simulink model "dual_arm_control"  (Simulink 7.8)
settings: Solver=ode1  StartTime=0.0  StopTime=inf  FixedStep=0.001  RelTol=1e-3
undefined symbols (not defined in the file): HIL
libraries: quarc_library x48, simulink x26, dspmtrx3 x5
(part 1 of 2)
settings Model: Creator=danso  LastModifiedBy=danso  SimulationMode=external  ExtModeTrigDuration=5000
settings SolverCC: PositivePriorityOrder=on
settings RTWCC: SystemTargetFile=quarc_win64.tlc  TemplateMakefile=quarc_default_tmf  Description=QUARC Win64 Target  ProcessScript=quarc_win64_make_rtw_hook
settings STFCustomTargetCC: TargetPreCompLibLocation=C:\PROGRA~3\QUARC\lib\2011b\win64\release  SystemTargetFile=quarc_win64.tlc
settings GRTTargetCC: TargetPreCompLibLocation=C:\PROGRA~3\QUARC\lib\2011b\win64\release  ParMdlRefBuildCompliant=off  CompOptLevelCompliant=off  ConcurrentExecutionCompliant=off  MatFileLogging=off  ExtMode=on  ExtModeMexFile=quarc_comm

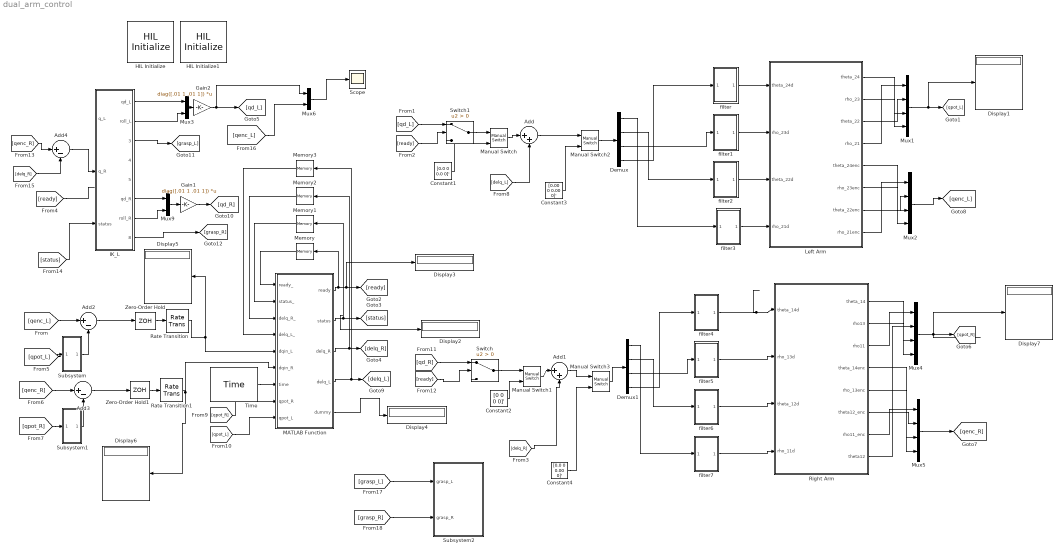
== system dual_arm_control ==
  Add : Sum  Inputs=|++
  Add1 : Sum  Inputs=|++
  Add2 : Sum  Inputs=|+-
  Add3 : Sum  Inputs=|+-
  Add4 : Sum  Inputs=|+-
  Constant1 : Constant  Value=[0.0 0 0.0 0]'
  Constant2 : Constant  Value=[0 0 0 0]'
  Constant3 : Constant  Value=[0.00 0 0.00 0]'
  Constant4 : Constant  Value=[0.0 0 0.00 0]'
  Demux : Demux
  Demux1 : Demux
  Display{1..7} (7 alike) : Display
  Gain1 : Gain  Gain=diag([.01 1 .01 1])  Multiplication=Matrix(K*u)
  Gain2 : Gain  Gain=diag([.01 1 .01 1])  Multiplication=Matrix(K*u)
  HIL Initialize : quarc_library/Data Acquisition/Generic/Configuration/HIL Initialize  Priority=-99  object_name=HIL-1  board_type=qpid_e  board_number=0  board_options=enc0_dir=0;enc0_filter=1;enc0_a=1;enc0_b=1;enc0_z=0;enc0_reload=0;enc1_dir=0;enc1_filter=1;enc1_a=1;enc1_b=1;enc1_z=0;enc1_reload=0;enc2_dir=0;enc2_filter=1;enc2_a=1;enc2_b=1;enc2_z=0;enc2_reload=0;enc3_dir=0;enc3_filter=1;enc3_a=1;enc3_b=1;enc3_z=0;enc3_reload=0;enc4_dir=0;enc4_filter=1;enc4_a=1;enc4_b=1;enc4_z=0;enc4_reload=0;enc5_dir=0;enc5_filter=1;enc5_a=1;enc5_b=1;enc5_z=0;enc5_reload=0;enc6_dir=0;enc6_filter=1;enc6_a=1;enc6_b=1;enc6_z=0;enc6_reload=0;enc7_dir=0;enc7_filter=1;enc7_a=1;enc7_b=1;enc7_z=0;enc7_reload=0;ext_int_polarity=0;fuse_polarity=0;convert_polarity=0;watchdog_polarity=0;ext_int_watchdog=0;fuse_watchdog=0;trig1_watchdog=0;watchdog_to_trig1=0;watchdog_to_trig2=0;counter_to_trig0=0;trigger_adcs=0;latch_on_adc=0;pwm_immediate=0  exclusive=off  active=off  hardware_clocks=[0:16]  clock_modes=[]  initial_clock_frequencies=[]  set_clock_params_at_start=off  set_clock_params_at_switch_in=off  set_clock_frequencies_at_start=off  set_clock_frequencies_at_switch_in=off  analog_input_channels=[0:7]  analog_input_maximums=10  analog_input_minimums=-10  set_analog_input_params_at_start=off  set_analog_input_params_at_switch_in=off  analog_output_channels=[0:7]  analog_output_maximums=10  analog_output_minimums=-10  initial_analog_outputs=[0]  final_analog_outputs=[0]  watchdog_analog_outputs=0  set_analog_output_params_at_start=off  set_analog_output_params_at_switch_in=off  set_analog_outputs_at_start=on  set_analog_outputs_at_switch_in=off  set_analog_outputs_at_terminate=on  set_analog_outputs_at_switch_out=off  set_analog_outputs_on_watchdog=off  digital_input_channels=[]  digital_output_channels=[0:31 46:47 40:45 55]  digital_output_configuration=[]  initial_digital_outputs=[1]  final_digital_outputs=[1]  watchdog_digital_outputs=[2]  set_digital_output_params_at_start=off  set_digital_output_params_at_switch_in=off  set_digital_outputs_at_start=on  set_digital_outputs_at_switch_in=off  set_digital_outputs_at_terminate=on  set_digital_outputs_at_switch_out=off  set_digital_outputs_on_watchdog=off  encoder_channels=[0:7]  quadrature=4  encoder_filter_frequency=40e6/1  initial_encoder_counts=[0]  set_encoder_params_at_start=on  set_encoder_params_at_switch_in=off  set_encoder_counts_at_start=on  set_encoder_counts_at_switch_in=off  pwm_channels=[0:7]  pwm_modes=0  pwm_frequency=40e6/4096  pwm_configuration=[0]  pwm_alignment=[0]  pwm_polarity=[1]  pwm_leading_deadband=[0]  pwm_trailing_deadband=[0]  initial_pwm_outputs=[0]  final_pwm_outputs=[0]  watchdog_pwm_outputs=[0]  set_pwm_params_at_start=on  set_pwm_params_at_switch_in=off  set_pwm_outputs_at_start=on  set_pwm_outputs_at_switch_in=off  set_pwm_outputs_at_terminate=on  set_pwm_outputs_at_switch_out=off  set_pwm_outputs_on_watchdog=off  other_output_channels=[]  initial_other_outputs=[]  final_other_outputs=[]  watchdog_other_outputs=[]  set_other_outputs_at_start=off  set_other_outputs_at_switch_in=off  set_other_outputs_at_terminate=off  set_other_outputs_at_switch_out=off  set_other_outputs_on_watchdog=off
  HIL Initialize1 : quarc_library/Data Acquisition/Generic/Configuration/HIL Initialize  Priority=-99  object_name=HIL-2  board_type=qpid  board_number=0  board_options=enc0_dir=0;enc0_filter=1;enc0_a=1;enc0_b=1;enc0_z=0;enc0_reload=0;enc1_dir=0;enc1_filter=1;enc1_a=1;enc1_b=1;enc1_z=0;enc1_reload=0;enc2_dir=0;enc2_filter=1;enc2_a=1;enc2_b=1;enc2_z=0;enc2_reload=0;enc3_dir=0;enc3_filter=1;enc3_a=1;enc3_b=1;enc3_z=0;enc3_reload=0;enc4_dir=0;enc4_filter=1;enc4_a=1;enc4_b=1;enc4_z=0;enc4_reload=0;enc5_dir=0;enc5_filter=1;enc5_a=1;enc5_b=1;enc5_z=0;enc5_reload=0;enc6_dir=0;enc6_filter=1;enc6_a=1;enc6_b=1;enc6_z=0;enc6_reload=0;enc7_dir=0;enc7_filter=1;enc7_a=1;enc7_b=1;enc7_z=0;enc7_reload=0;ext_int_polarity=0;fuse_polarity=0;convert_polarity=0;watchdog_polarity=0;ext_int_watchdog=0;fuse_watchdog=0;trig1_watchdog=0;watchdog_to_trig1=0;watchdog_to_trig2=0;counter_to_trig0=0;trigger_adcs=0;latch_on_adc=0;pwm_immediate=0  exclusive=off  active=off  hardware_clocks=[0:16]  clock_modes=[]  initial_clock_frequencies=[]  set_clock_params_at_start=off  set_clock_params_at_switch_in=off  set_clock_frequencies_at_start=off  set_clock_frequencies_at_switch_in=off  analog_input_channels=[0:7]  analog_input_maximums=10  analog_input_minimums=-10  set_analog_input_params_at_start=off  set_analog_input_params_at_switch_in=off  analog_output_channels=[0:7]  analog_output_maximums=10  analog_output_minimums=-10  initial_analog_outputs=[0]  final_analog_outputs=[0]  watchdog_analog_outputs=0  set_analog_output_params_at_start=off  set_analog_output_params_at_switch_in=off  set_analog_outputs_at_start=on  set_analog_outputs_at_switch_in=off  set_analog_outputs_at_terminate=on  set_analog_outputs_at_switch_out=off  set_analog_outputs_on_watchdog=off  digital_input_channels=[48:55]  digital_output_channels=[]  digital_output_configuration=[]  initial_digital_outputs=[1]  final_digital_outputs=[1]  watchdog_digital_outputs=[2]  set_digital_output_params_at_start=off  set_digital_output_params_at_switch_in=off  set_digital_outputs_at_start=on  set_digital_outputs_at_switch_in=off  set_digital_outputs_at_terminate=on  set_digital_outputs_at_switch_out=off  set_digital_outputs_on_watchdog=off  encoder_channels=[0:7]  quadrature=[4]  encoder_filter_frequency=40e6/1  initial_encoder_counts=[0]  set_encoder_params_at_start=on  set_encoder_params_at_switch_in=off  set_encoder_counts_at_start=on  set_encoder_counts_at_switch_in=off  pwm_channels=[0:7]  pwm_modes=0  pwm_frequency=40e6/4096  pwm_configuration=[0]  pwm_alignment=[0]  pwm_polarity=[1]  pwm_leading_deadband=[0]  pwm_trailing_deadband=[0]  initial_pwm_outputs=[0]  final_pwm_outputs=[0]  watchdog_pwm_outputs=[0]  set_pwm_params_at_start=on  set_pwm_params_at_switch_in=off  set_pwm_outputs_at_start=on  set_pwm_outputs_at_switch_in=off  set_pwm_outputs_at_terminate=on  set_pwm_outputs_at_switch_out=off  set_pwm_outputs_on_watchdog=off  other_output_channels=[]  initial_other_outputs=[]  final_other_outputs=[]  watchdog_other_outputs=[]  set_other_outputs_at_start=off  set_other_outputs_at_switch_in=off  set_other_outputs_at_terminate=off  set_other_outputs_at_switch_out=off  set_other_outputs_on_watchdog=off
  IK_L : Subsystem
  Left Arm : Subsystem
  MATLAB Function : MATLAB Function  TreatAsAtomicUnit=on
  Manual Switch{,1..3} (4 alike) : simulink/Signal Routing/Manual Switch  sw=1  action=0  varsize=off
  Memory : Memory
  Memory1 : Memory
  Memory2 : Memory  X0=[0 0 0 0 ]'
  Memory3 : Memory  X0=[0 0 0 0]'
  Mux{1..2,4..5} (4 alike) : Mux
  Mux3 : Mux  Inputs=[3 1]
  Mux6 : Mux  Inputs=2
  Mux9 : Mux  Inputs=[3 1]
  Rate Transition : RateTransition
  Rate Transition1 : RateTransition
  Right Arm : Subsystem
  Scope : Scope
      settings: YMin=-1.5  YMax=7.5
  Subsystem : Subsystem
  Subsystem1 : Subsystem
  Subsystem2 : Subsystem
  Switch : Switch  Criteria=u2 > Threshold
  Switch1 : Switch  Criteria=u2 > Threshold
  Time : quarc_library/Sources/Time/Time  sample_time=qc_get_step_size
  Zero-Order Hold : ZeroOrderHold  SampleTime=2
  Zero-Order Hold1 : ZeroOrderHold  SampleTime=2
  filter : Subsystem
  filter1 : Subsystem
  filter2 : Subsystem
  filter3 : Subsystem
  filter4 : Subsystem
  filter5 : Subsystem
  filter6 : Subsystem
  filter7 : Subsystem
  wires:
  IK_L/1(qd_L) -> Mux3/1
  Mux3/1 -> Gain2/1
  IK_L/2(roll_L) -> Mux3/2
  Mux9/1 -> Gain1/1
  IK_L/6(qd_R) -> Mux9/1
  IK_L/7(roll_R) -> Mux9/2
  [ready] -> ?
  ? -> IK_L/1(q_L)
  Demux/3 -> filter1/1(In1)
  Demux/4 -> filter/1(In1)
  Demux/2 -> filter2/1(In1)
  filter3/1(Out1) -> Left Arm/4(rho_21d)
  filter2/1(Out1) -> Left Arm/3(theta_22d)
  filter1/1(Out1) -> Left Arm/2(rho_23d)
  filter/1(Out1) -> Left Arm/1(theta_24d)
  Demux/1 -> filter3/1(In1)
  filter4/1(Out1) -> Right Arm/1(theta_14d)
  filter5/1(Out1) -> Right Arm/2(rho_13d)
  filter6/1(Out1) -> Right Arm/3(theta_12d)
  filter7/1(Out1) -> Right Arm/4(rho_11d)
  Mux5/1 -> [qenc_R]
  Mux4/1 -> [qpot_R], Display7/1
  Right Arm/3(rho11) -> Mux4/1
  Right Arm/2(rho13) -> Mux4/3
  Right Arm/1(theta_14) -> Mux4/4
  Right Arm/7(rho11_enc) -> Mux5/1
  Right Arm/6(theta12_enc) -> Mux5/2
  Right Arm/5(rho_13enc) -> Mux5/3
  Right Arm/4(theta_14enc) -> Mux5/4
  Left Arm/4(rho_21) -> Mux1/1
  Left Arm/3(theta_22) -> Mux1/2
  Left Arm/2(rho_23) -> Mux1/3
  Left Arm/1(theta_24) -> Mux1/4
  Left Arm/8(rho_21enc) -> Mux2/1
  Left Arm/7(theta_22enc) -> Mux2/2
  Left Arm/6(rho_23enc) -> Mux2/3
  Left Arm/5(theta_24enc) -> Mux2/4
  Demux1/4 -> filter4/1(In1)
  Demux1/2 -> filter6/1(In1)
  Demux1/1 -> filter7/1(In1)
  Mux1/1 -> [qpot_L], Display1/1
  Mux2/1 -> [qenc_L]
  Right Arm/8(theta12) -> Mux4/2
  Demux1/3 -> filter5/1(In1)
  Gain2/1 -> Mux6/1, [qd_L]
  Gain1/1 -> [qd_R]
  Constant2/1 -> Manual Switch1/2
  Constant1/1 -> Manual Switch/2
  [delq_L] -> Add/2
  [delq_R] -> Add1/2
  MATLAB Function/1(ready) -> Memory/1, [ready], Display3/1
  MATLAB Function/2(status) -> [status], Memory1/1, Display2/1
  Memory/1 -> MATLAB Function/1(ready_)
  Memory1/1 -> MATLAB Function/2(status_)
  Zero-Order Hold/1 -> Rate Transition/1
  [qenc_L] -> Add2/1
  [qpot_L] -> Subsystem/1(In1)
  Add2/1 -> Zero-Order Hold/1
  Rate Transition/1 -> Display5/1, MATLAB Function/5(dqin_L)
  Zero-Order Hold1/1 -> Rate Transition1/1
  [qenc_R] -> Add3/1
  [qpot_R] -> Subsystem1/1(In1)
  Add3/1 -> Zero-Order Hold1/1
  Rate Transition1/1 -> Display6/1, MATLAB Function/6(dqin_R)
  MATLAB Function/3(delq_R) -> [delq_R], Memory2/1
  MATLAB Function/4(delq_L) -> [delq_L], Memory3/1
  Time/1 -> MATLAB Function/7(time)
  MATLAB Function/5(dummy) -> Display4/1
  [qpot_R] -> MATLAB Function/8(qpot_R)
  [qpot_L] -> MATLAB Function/9(qpot_L)
  Memory2/1 -> MATLAB Function/3(delq_R_)
  Memory3/1 -> MATLAB Function/4(delq_L_)
  [ready] -> Switch/2
  Subsystem1/1(Out1) -> Add3/2
  [qd_R] -> Switch/1
  [status] -> IK_L/3(status)
  [qenc_R] -> Add4/1
  [delq_R] -> Add4/2
  Add4/1 -> IK_L/2(q_R)
  Subsystem/1(Out1) -> Add2/2
  Switch1/1 -> Manual Switch/1
  [qd_L] -> Switch1/1
  [ready] -> Switch1/2
  [qenc_L] -> Mux6/2
  Mux6/1 -> Scope/1
  Manual Switch/1 -> Add/1
  Manual Switch1/1 -> Add1/1
  Switch/1 -> Manual Switch1/1
  [grasp_L] -> Subsystem2/1(grasp_L)
  [grasp_R] -> Subsystem2/2(grasp_R)
  IK_L/3(grasp_L) -> [grasp_L]
  IK_L/8(grasp_R) -> [grasp_R]
  Manual Switch2/1 -> Demux/1
  Constant3/1 -> Manual Switch2/2
  Add/1 -> Manual Switch2/1
  Manual Switch3/1 -> Demux1/1
  Add1/1 -> Manual Switch3/1
  Constant4/1 -> Manual Switch3/2

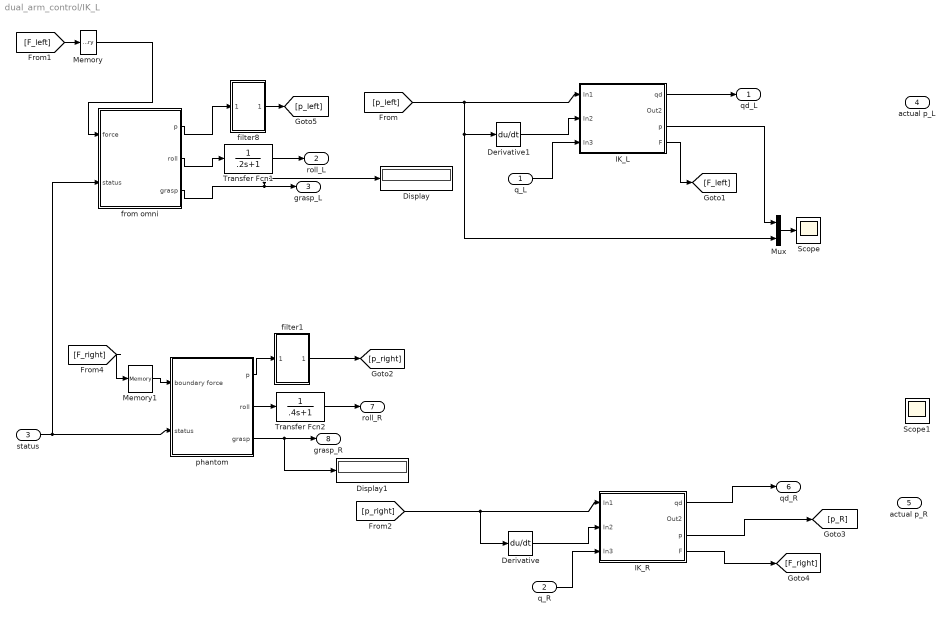
== system dual_arm_control/IK_L ==
  q_L : Inport
  q_R : Inport  Port=2
  status : Inport  Port=3
  Derivative : Derivative
  Derivative1 : Derivative
  Display : Display
  Display1 : Display
  IK_L : Subsystem
  IK_R : Subsystem
  Memory : Memory
  Memory1 : Memory
  Mux : Mux  Inputs=2
  Scope : Scope
      settings: YMin=-2  YMax=5.5
  Scope1 : Scope
      settings: YMin=-1.5  YMax=4  SaveName=ScopeData5
  Transfer Fcn1 : TransferFcn  Denominator=[.2 1]
  Transfer Fcn2 : TransferFcn  Denominator=[.4 1]
  filter1 : Subsystem
  filter8 : Subsystem
  from omni : Subsystem
  phantom : Subsystem
  qd_L : Outport
  roll_L : Outport  Port=2
  grasp_L : Outport  Port=3
  actual p_L : Outport  Port=4
  actual p_R : Outport  Port=5
  qd_R : Outport  Port=6
  roll_R : Outport  Port=7
  grasp_R : Outport  Port=8
  wires:
  from omni/1(p) -> filter8/1(In1)
  [F_left] -> Memory/1
  from omni/3(grasp) -> Display/1, grasp_L/1
  [p_left] -> Derivative1/1, Mux/2, IK_L/1(In1)
  Derivative1/1 -> IK_L/2(In2)
  IK_L/1(qd) -> qd_L/1
  IK_L/4(F) -> [F_left]
  Memory/1 -> from omni/1(force)
  phantom/1(p) -> filter1/1(In1)
  [F_right] -> Memory1/1
  phantom/2(roll) -> Transfer Fcn2/1
  phantom/3(grasp) -> grasp_R/1, Display1/1
  [p_right] -> Derivative/1, IK_R/1(In1)
  IK_R/4(F) -> [F_right]
  IK_R/1(qd) -> qd_R/1
  Derivative/1 -> IK_R/2(In2)
  from omni/2(roll) -> Transfer Fcn1/1
  Memory1/1 -> phantom/1(boundary force)
  filter1/1(Out1) -> [p_right]
  Transfer Fcn2/1 -> roll_R/1
  q_L/1 -> IK_L/3(In3)
  Mux/1 -> Scope/1
  IK_L/3(p) -> Mux/1
  status/1 -> phantom/2(status), from omni/2(status)
  IK_R/3(p) -> [p_R]
  q_R/1 -> IK_R/3(In3)
  Transfer Fcn1/1 -> roll_L/1
  filter8/1(Out1) -> [p_left]

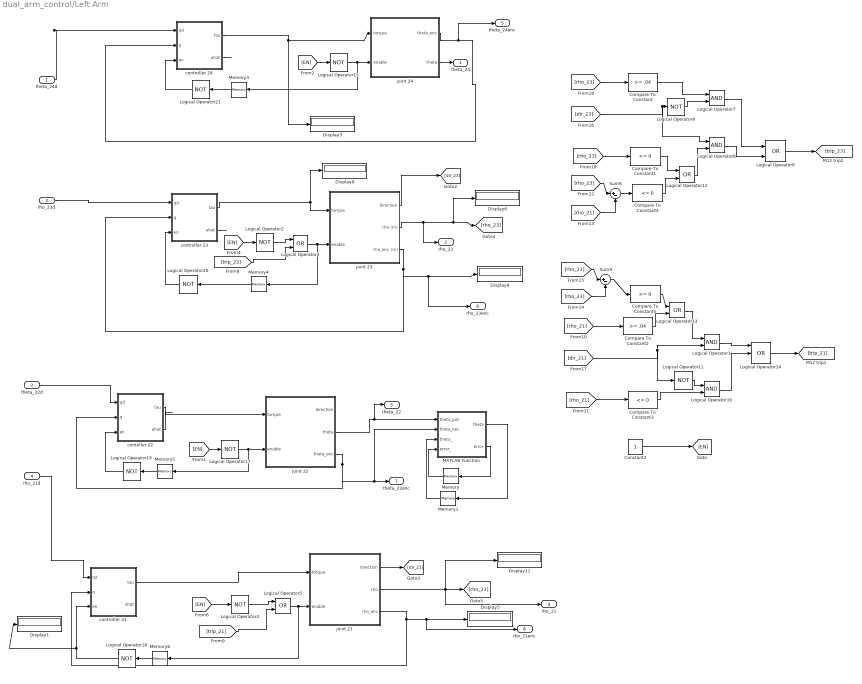
== system dual_arm_control/Left Arm ==
  theta_24d : Inport
  rho_23d : Inport  Port=2
  theta_22d : Inport  Port=3
  rho_21d : Inport  Port=4
  Compare To Constant : simulink/Logic and Bit Operations/Compare To Constant  relop=>=  const=.04  OutDataTypeStr=uint8
  Compare To Constant1 : simulink/Logic and Bit Operations/Compare To Constant  relop=<=  const=0  OutDataTypeStr=uint8
  Compare To Constant2 : simulink/Logic and Bit Operations/Compare To Constant  relop=>=  const=.04  OutDataTypeStr=uint8
  Compare To Constant3 : simulink/Logic and Bit Operations/Compare To Constant  relop=<=  const=0  OutDataTypeStr=uint8
  Compare To Constant4 : simulink/Logic and Bit Operations/Compare To Constant  relop=<=  const=0  OutDataTypeStr=uint8
  Compare To Constant5 : simulink/Logic and Bit Operations/Compare To Constant  relop=>=  const=0  OutDataTypeStr=uint8
  Constant2 : Constant
  Display{1,3,5..6,8..9,11} (7 alike) : Display
  Logical Operator{1,7..8,10} (4 alike) : Logic  AllPortsSameDT=off  OutDataTypeStr=boolean
  Logical Operator{2,4,9,11,15,17..21} (10 alike) : Logic  Operator=NOT  AllPortsSameDT=off  OutDataTypeStr=boolean
  Logical Operator{3,5..6,12..13} (5 alike) : Logic  Operator=OR  AllPortsSameDT=off  OutDataTypeStr=boolean
  Logical Operator14 : Logic  Operator=OR  Inputs=3  AllPortsSameDT=off  OutDataTypeStr=boolean
  MATLAB Function : MATLAB Function  TreatAsAtomicUnit=on
  Memory{,1,3..6} (6 alike) : Memory
  Sum8 : Sum  Inputs=|+-
  Sum9 : Sum  Inputs=|+-
  contoller 22 : Subsystem
  controller 21 : Subsystem
  controller 23 : Subsystem
  controller 24 : Subsystem
  joint 21 : Subsystem
  joint 22 : Subsystem
  joint 23 : Subsystem
  joint 24 : Subsystem
  theta_24 : Outport
  rho_23 : Outport  Port=2
  theta_22 : Outport  Port=3
  rho_21 : Outport  Port=4
  theta_24enc : Outport  Port=5
  rho_23enc : Outport  Port=6
  theta_22enc : Outport  Port=7
  rho_21enc : Outport  Port=8
  wires:
  Memory6/1 -> Logical Operator18/1
  Memory5/1 -> Logical Operator19/1
  [EN] -> Logical Operator4/1
  Logical Operator4/1 -> Logical Operator5/1
  [trip_21] -> Logical Operator5/2
  joint 21/2(rho) -> [rho_21], Display11/1, rho_21/1
  joint 22/3(theta_enc) -> contoller 22/2(q), theta_22enc/1, MATLAB Function/2(theta_enc)
  contoller 22/1(tau) -> joint 22/1(torque)
  Logical Operator17/1 -> joint 22/2(enable), Memory5/1
  [EN] -> Logical Operator17/1
  joint 21/1(direction) -> [dir_21]
  Logical Operator5/1 -> joint 21/2(enable), Memory6/1
  joint 21/3(rho_enc) -> Display5/1, rho_21enc/1, controller 21/2(q)
  joint 24/1(theta_enc) -> controller 24/2(q), theta_24enc/1
  controller 24/1(tau) -> Display3/1, joint 24/1(torque)
  [EN] -> Logical Operator2/1
  [trip_23] -> Logical Operator3/2
  Logical Operator2/1 -> Logical Operator3/1
  joint 23/1(direction) -> [dir_23]
  Logical Operator3/1 -> joint 23/2(enable), Memory4/1
  theta_24d/1 -> controller 24/1(qd)
  joint 23/2(rho (m)) -> [rho_23], Display6/1, rho_23/1
  joint 23/3(rho_enc (m)) -> controller 23/2(q), Display8/1, rho_23enc/1
  controller 23/1(tau) -> Display9/1, joint 23/1(torque)
  [EN] -> Logical Operator15/1
  Logical Operator15/1 -> joint 24/2(enable), Memory3/1
  Memory3/1 -> Logical Operator21/1
  Memory4/1 -> Logical Operator20/1
  controller 24/2(ahat) -> ?
  joint 24/2(theta) -> theta_24/1
  rho_23d/1 -> controller 23/1(qd)
  controller 23/2(ahat) -> ?
  theta_22d/1 -> contoller 22/1(qd)
  contoller 22/2(ahat) -> ?
  rho_21d/1 -> controller 21/1(qd)
  Logical Operator6/1 -> [trip_23]
  [dir_23] -> Logical Operator8/1, Logical Operator9/1
  Compare To Constant/1 -> Logical Operator7/1
  [rho_23] -> Compare To Constant1/1
  Logical Operator7/1 -> Logical Operator6/1
  Logical Operator8/1 -> Logical Operator6/2
  Logical Operator9/1 -> Logical Operator7/2
  [rho_23] -> Sum8/1
  [rho_21] -> Sum8/2
  Sum8/1 -> Compare To Constant4/1
  Compare To Constant4/1 -> Logical Operator12/2
  Compare To Constant1/1 -> Logical Operator12/1
  Logical Operator12/1 -> Logical Operator8/2
  [dir_21] -> Logical Operator11/1, Logical Operator1/2
  Compare To Constant3/1 -> Logical Operator10/2
  Logical Operator11/1 -> Logical Operator10/1
  [rho_21] -> Compare To Constant2/1
  [rho_21] -> Compare To Constant3/1
  Logical Operator13/1 -> Logical Operator1/1
  Compare To Constant2/1 -> Logical Operator13/2
  Sum9/1 -> Compare To Constant5/1
  [rho_21] -> Sum9/1
  [rho_23] -> Sum9/2
  Compare To Constant5/1 -> Logical Operator13/1
  Logical Operator1/1 -> Logical Operator14/1
  Logical Operator10/1 -> Logical Operator14/2
  Logical Operator14/1 -> [trip_21]
  Constant2/1 -> [EN]
  controller 21/1(tau) -> joint 21/1(torque)
  Logical Operator18/1 -> controller 21/3(en), Display1/1
  Logical Operator19/1 -> contoller 22/3(en)
  Logical Operator20/1 -> controller 23/3(en)
  Logical Operator21/1 -> controller 24/3(en)
  [rho_23] -> Compare To Constant/1
  Memory/1 -> MATLAB Function/4(error_)
  MATLAB Function/2(error) -> Memory/1
  MATLAB Function/1(theta) -> Memory1/1
  Memory1/1 -> MATLAB Function/3(theta_)
  joint 22/2(theta) -> MATLAB Function/1(theta_pot), theta_22/1

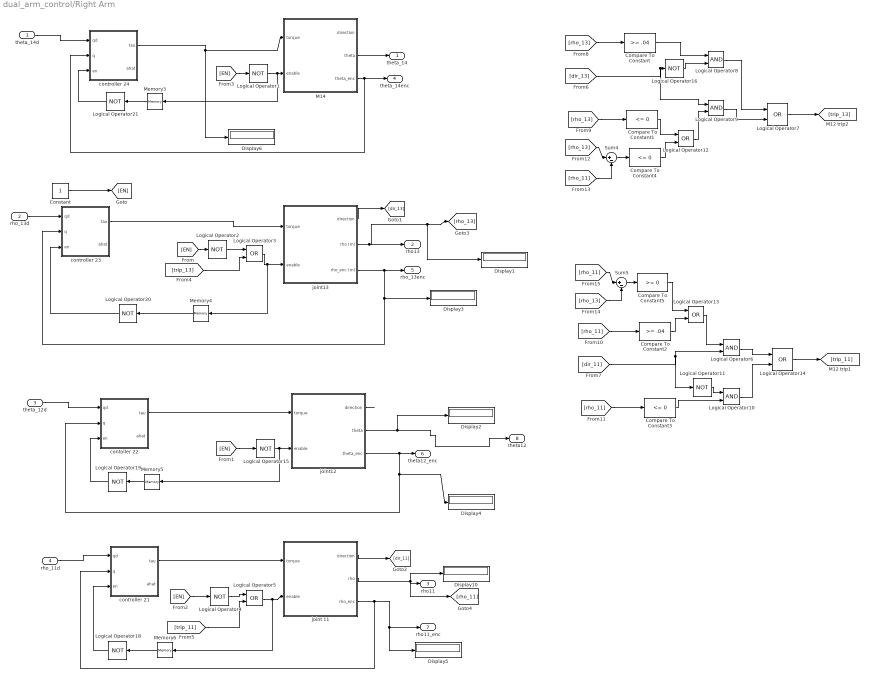
== system dual_arm_control/Right Arm ==
  theta_14d : Inport
  rho_13d : Inport  Port=2
  theta_12d : Inport  Port=3
  rho_11d : Inport  Port=4
  Compare To Constant : simulink/Logic and Bit Operations/Compare To Constant  relop=>=  const=.04  OutDataTypeStr=uint8
  Compare To Constant1 : simulink/Logic and Bit Operations/Compare To Constant  relop=<=  const=0  OutDataTypeStr=uint8
  Compare To Constant2 : simulink/Logic and Bit Operations/Compare To Constant  relop=>=  const=.04  OutDataTypeStr=uint8
  Compare To Constant3 : simulink/Logic and Bit Operations/Compare To Constant  relop=<=  const=0  OutDataTypeStr=uint8
  Compare To Constant4 : simulink/Logic and Bit Operations/Compare To Constant  relop=<=  const=0  OutDataTypeStr=uint8
  Compare To Constant5 : simulink/Logic and Bit Operations/Compare To Constant  relop=>=  const=0  OutDataTypeStr=uint8
  Constant : Constant
  Display{1..6,10} (7 alike) : Display
  Logical Operator{1..2,4,11,15..16,18..21} (10 alike) : Logic  Operator=NOT  AllPortsSameDT=off  OutDataTypeStr=boolean
  Logical Operator{6,8..10} (4 alike) : Logic  AllPortsSameDT=off  OutDataTypeStr=boolean
  Logical Operator{3,5,7,12..14} (6 alike) : Logic  Operator=OR  AllPortsSameDT=off  OutDataTypeStr=boolean
  M14 : Subsystem
  Memory{3..6} (4 alike) : Memory
  Sum4 : Sum  Inputs=|+-
  Sum5 : Sum  Inputs=|+-
  contoller 22 : Subsystem
  controller 21 : Subsystem
  controller 23 : Subsystem
  controller 24 : Subsystem
  joint 11 : Subsystem
  joint12 : Subsystem
  joint13 : Subsystem
  theta_14 : Outport
  rho13 : Outport  Port=2
  rho11 : Outport  Port=3
  theta_14enc : Outport  Port=4
  rho_13enc : Outport  Port=5
  theta12_enc : Outport  Port=6
  rho11_enc : Outport  Port=7
  theta12 : Outport  Port=8
  wires:
  Constant/1 -> [EN]
  [EN] -> Logical Operator2/1
  Logical Operator3/1 -> joint13/2(enable), Memory4/1
  [trip_13] -> Logical Operator3/2
  Logical Operator2/1 -> Logical Operator3/1
  joint13/1(direction) -> [dir_13]
  controller 23/1(tau) -> joint13/1(torque)
  joint13/2(rho (m)) -> rho13/1, [rho_13], Display1/1
  joint13/3(rho_enc (m)) -> Display3/1, controller 23/2(q), rho_13enc/1
  Memory4/1 -> Logical Operator20/1
  Logical Operator20/1 -> controller 23/3(en)
  [EN] -> Logical Operator15/1
  Logical Operator15/1 -> joint12/2(enable), Memory5/1
  joint12/3(theta_enc) -> contoller 22/2(q), Display4/1, theta12_enc/1
  joint12/2(theta) -> Display2/1, theta12/1
  Memory5/1 -> Logical Operator19/1
  Logical Operator19/1 -> contoller 22/3(en)
  contoller 22/1(tau) -> joint12/1(torque)
  [trip_11] -> Logical Operator5/2
  Logical Operator4/1 -> Logical Operator5/1
  [EN] -> Logical Operator4/1
  Logical Operator5/1 -> joint 11/2(enable), Memory6/1
  joint 11/1(direction) -> [dir_11]
  joint 11/3(rho_enc) -> Display5/1, rho11_enc/1, controller 21/2(q)
  joint 11/2(rho) -> rho11/1, Display10/1, [rho_11]
  controller 21/1(tau) -> joint 11/1(torque)
  Memory6/1 -> Logical Operator18/1
  Logical Operator18/1 -> controller 21/3(en)
  M14/2(theta) -> theta_14/1
  controller 24/1(tau) -> Display6/1, M14/1(torque)
  [EN] -> Logical Operator1/1
  Logical Operator1/1 -> Memory3/1, M14/2(enable)
  Memory3/1 -> Logical Operator21/1
  M14/3(theta_enc) -> controller 24/2(q), theta_14enc/1
  Logical Operator21/1 -> controller 24/3(en)
  theta_14d/1 -> controller 24/1(qd)
  rho_13d/1 -> controller 23/1(qd)
  theta_12d/1 -> contoller 22/1(qd)
  rho_11d/1 -> controller 21/1(qd)
  joint12/1(direction) -> ?
  Logical Operator7/1 -> [trip_13]
  [dir_13] -> Logical Operator9/1, Logical Operator16/1
  Compare To Constant/1 -> Logical Operator8/1
  [rho_13] -> Compare To Constant/1
  [rho_13] -> Compare To Constant1/1
  [dir_11] -> Logical Operator11/1, Logical Operator6/2
  Compare To Constant3/1 -> Logical Operator10/2
  Logical Operator11/1 -> Logical Operator10/1
  [rho_11] -> Compare To Constant2/1
  [rho_11] -> Compare To Constant3/1
  Logical Operator8/1 -> Logical Operator7/1
  Logical Operator9/1 -> Logical Operator7/2
  Logical Operator16/1 -> Logical Operator8/2
  [rho_13] -> Sum4/1
  [rho_11] -> Sum4/2
  Sum4/1 -> Compare To Constant4/1
  Compare To Constant4/1 -> Logical Operator12/2
  Compare To Constant1/1 -> Logical Operator12/1
  Logical Operator12/1 -> Logical Operator9/2
  Logical Operator13/1 -> Logical Operator6/1
  Compare To Constant2/1 -> Logical Operator13/2
  Sum5/1 -> Compare To Constant5/1
  [rho_11] -> Sum5/1
  [rho_13] -> Sum5/2
  Compare To Constant5/1 -> Logical Operator13/1
  Logical Operator6/1 -> Logical Operator14/1
  Logical Operator10/1 -> Logical Operator14/2
  Logical Operator14/1 -> [trip_11]

== system dual_arm_control/Subsystem ==
  In1 : Inport
  Demux2 : Demux
  Mux6 : Mux
  Transfer Fcn{,1..3} (4 alike) : TransferFcn  Denominator=[1 1]
  Out1 : Outport
  wires:
  Transfer Fcn3/1 -> Mux6/1
  Transfer Fcn2/1 -> Mux6/2
  Transfer Fcn1/1 -> Mux6/3
  Transfer Fcn/1 -> Mux6/4
  Demux2/1 -> Transfer Fcn3/1
  Demux2/2 -> Transfer Fcn2/1
  Demux2/3 -> Transfer Fcn1/1
  Demux2/4 -> Transfer Fcn/1
  Mux6/1 -> Out1/1
  In1/1 -> Demux2/1

== system dual_arm_control/Subsystem1 ==
  In1 : Inport
  Demux2 : Demux
  Mux6 : Mux
  Transfer Fcn{,1..3} (4 alike) : TransferFcn  Denominator=[1 1]
  Out1 : Outport
  wires:
  Transfer Fcn3/1 -> Mux6/1
  Transfer Fcn2/1 -> Mux6/2
  Transfer Fcn1/1 -> Mux6/3
  Transfer Fcn/1 -> Mux6/4
  Demux2/1 -> Transfer Fcn3/1
  Demux2/2 -> Transfer Fcn2/1
  Demux2/3 -> Transfer Fcn1/1
  Demux2/4 -> Transfer Fcn/1
  Mux6/1 -> Out1/1
  In1/1 -> Demux2/1

== system dual_arm_control/Subsystem2 ==
  grasp_L : Inport
  grasp_R : Inport  Port=2
  Constant : Constant  Value=9.2
  Constant1 : Constant  Value=6
  Constant2 : Constant  Value=9.5
  Constant3 : Constant  Value=6.5
  Demux : Demux  Outputs=3
  Demux1 : Demux  Outputs=3
  Display3 : Display
  Display5 : Display
  E1-1 : Subsystem
  E1-2 : Subsystem
  MATLAB Function : MATLAB Function  TreatAsAtomicUnit=on
  MATLAB Function1 : MATLAB Function  TreatAsAtomicUnit=on
  Mux : Mux  Inputs=3
  Mux1 : Mux  Inputs=3
  Subsystem : Subsystem
  wires:
  E1-1/1(Out1) -> Display3/1, MATLAB Function/2(pos)
  E1-2/1(Out1) -> Display5/1, MATLAB Function1/2(pos)
  MATLAB Function/1(dir) -> Mux/1
  MATLAB Function/2(en) -> Mux/2
  MATLAB Function/3(pwm) -> Mux/3
  MATLAB Function1/1(dir) -> Mux1/1
  MATLAB Function1/2(en) -> Mux1/2
  MATLAB Function1/3(pwm) -> Mux1/3
  Mux/1 -> Demux/1
  Demux/1 -> Subsystem/1(DIR_1)
  Demux/2 -> Subsystem/2(EN_1)
  Demux/3 -> Subsystem/3(PWM_1)
  Mux1/1 -> Demux1/1
  Demux1/1 -> Subsystem/4(DIR_2)
  Demux1/2 -> Subsystem/5(EN_2)
  Demux1/3 -> Subsystem/6(PWM_2)
  grasp_L/1 -> MATLAB Function/1(u)
  grasp_R/1 -> MATLAB Function1/1(u)
  Constant/1 -> MATLAB Function/3(pmax)
  Constant1/1 -> MATLAB Function/4(pmin)
  Constant2/1 -> MATLAB Function1/3(pmax)
  Constant3/1 -> MATLAB Function1/4(pmin)

== system dual_arm_control/filter ==
  In1 : Inport
  Memory : Memory
  filter : MATLAB Function  TreatAsAtomicUnit=on
  Out1 : Outport
  wires:
  filter/1(y) -> Memory/1, Out1/1
  Memory/1 -> filter/2(u_)
  In1/1 -> filter/1(u)

== system dual_arm_control/filter1 ==
  In1 : Inport
  Memory : Memory
  filter : MATLAB Function  TreatAsAtomicUnit=on
  Out1 : Outport
  wires:
  filter/1(y) -> Memory/1, Out1/1
  Memory/1 -> filter/2(u_)
  In1/1 -> filter/1(u)

== system dual_arm_control/filter2 ==
  In1 : Inport
  Memory : Memory
  filter : MATLAB Function  TreatAsAtomicUnit=on
  Out1 : Outport
  wires:
  filter/1(y) -> Memory/1, Out1/1
  Memory/1 -> filter/2(u_)
  In1/1 -> filter/1(u)

== system dual_arm_control/filter3 ==
  In1 : Inport
  Memory : Memory
  filter : MATLAB Function  TreatAsAtomicUnit=on
  Out1 : Outport
  wires:
  filter/1(y) -> Memory/1, Out1/1
  Memory/1 -> filter/2(u_)
  In1/1 -> filter/1(u)

== system dual_arm_control/filter4 ==
  In1 : Inport
  Memory : Memory
  filter : MATLAB Function  TreatAsAtomicUnit=on
  Out1 : Outport
  wires:
  filter/1(y) -> Memory/1, Out1/1
  Memory/1 -> filter/2(u_)
  In1/1 -> filter/1(u)

== system dual_arm_control/filter5 ==
  In1 : Inport
  Memory : Memory
  filter : MATLAB Function  TreatAsAtomicUnit=on
  Out1 : Outport
  wires:
  filter/1(y) -> Memory/1, Out1/1
  Memory/1 -> filter/2(u_)
  In1/1 -> filter/1(u)

== system dual_arm_control/filter6 ==
  In1 : Inport
  Memory : Memory
  filter : MATLAB Function  TreatAsAtomicUnit=on
  Out1 : Outport
  wires:
  filter/1(y) -> Memory/1, Out1/1
  Memory/1 -> filter/2(u_)
  In1/1 -> filter/1(u)

== system dual_arm_control/filter7 ==
  In1 : Inport
  Memory : Memory
  filter : MATLAB Function  TreatAsAtomicUnit=on
  Out1 : Outport
  wires:
  filter/1(y) -> Memory/1, Out1/1
  Memory/1 -> filter/2(u_)
  In1/1 -> filter/1(u)

== system dual_arm_control/IK_L/IK_L ==
  In1 : Inport
  In2 : Inport  Port=2
  In3 : Inport  Port=3
  Display : Display
  IK : MATLAB Function  TreatAsAtomicUnit=on
  Integrator : Integrator
  Memory1 : Memory  X0=[0 0 0]'
  Memory3 : Memory
  Memory4 : Memory
  qd : Outport
  Out2 : Outport  Port=2
  p : Outport  Port=3
  F : Outport  Port=4
  wires:
  IK/1(q) -> Memory1/1
  IK/5(F) -> F/1
  IK/6(k) -> Memory3/1
  Memory3/1 -> IK/4(k_)
  IK/3(qdot) -> Integrator/1
  IK/2(qm) -> qd/1, Display/1
  IK/7(r) -> Memory4/1
  Memory4/1 -> IK/5(r_)
  In1/1 -> IK/2(pd)
  Integrator/1 -> Out2/1
  In2/1 -> IK/3(pd_d)
  IK/4(p) -> p/1
  Memory1/1 -> IK/1(q_)

== system dual_arm_control/IK_L/IK_R ==
  In1 : Inport
  In2 : Inport  Port=2
  In3 : Inport  Port=3
  Display : Display
  IK : MATLAB Function  TreatAsAtomicUnit=on
  Integrator : Integrator
  Memory1 : Memory  X0=[0 0 0]'
  Memory3 : Memory
  Memory4 : Memory
  qd : Outport
  Out2 : Outport  Port=2
  p : Outport  Port=3
  F : Outport  Port=4
  wires:
  IK/1(q) -> Memory1/1
  IK/5(F) -> F/1
  IK/6(k) -> Memory3/1
  Memory3/1 -> IK/4(k_)
  IK/3(qdot) -> Integrator/1
  IK/2(qm) -> qd/1, Display/1
  IK/7(r) -> Memory4/1
  Memory4/1 -> IK/5(r_)
  In1/1 -> IK/2(pd)
  Integrator/1 -> Out2/1
  In2/1 -> IK/3(pd_d)
  IK/4(p) -> p/1
  Memory1/1 -> IK/1(q_)

== system dual_arm_control/IK_L/filter1 ==
  In1 : Inport
  Demux : Demux  Outputs=3
  Mux : Mux  Inputs=3
  Transfer Fcn : TransferFcn  Denominator=[.4 1]
  Transfer Fcn1 : TransferFcn  Denominator=[.4 1]
  Transfer Fcn2 : TransferFcn  Denominator=[.4 1]
  Out1 : Outport
  wires:
  Transfer Fcn/1 -> Mux/1
  Transfer Fcn1/1 -> Mux/2
  Transfer Fcn2/1 -> Mux/3
  Demux/1 -> Transfer Fcn/1
  Demux/2 -> Transfer Fcn1/1
  Demux/3 -> Transfer Fcn2/1
  Mux/1 -> Out1/1
  In1/1 -> Demux/1

== system dual_arm_control/IK_L/filter8 ==
  In1 : Inport
  Demux : Demux  Outputs=3
  Mux : Mux  Inputs=3
  Transfer Fcn : TransferFcn  Denominator=[.5 1]
  Transfer Fcn1 : TransferFcn  Denominator=[.5 1]
  Transfer Fcn2 : TransferFcn  Denominator=[.5 1]
  Out1 : Outport
  wires:
  Transfer Fcn/1 -> Mux/1
  Transfer Fcn1/1 -> Mux/2
  Transfer Fcn2/1 -> Mux/3
  Demux/1 -> Transfer Fcn/1
  Demux/2 -> Transfer Fcn1/1
  Demux/3 -> Transfer Fcn2/1
  Mux/1 -> Out1/1
  In1/1 -> Demux/1

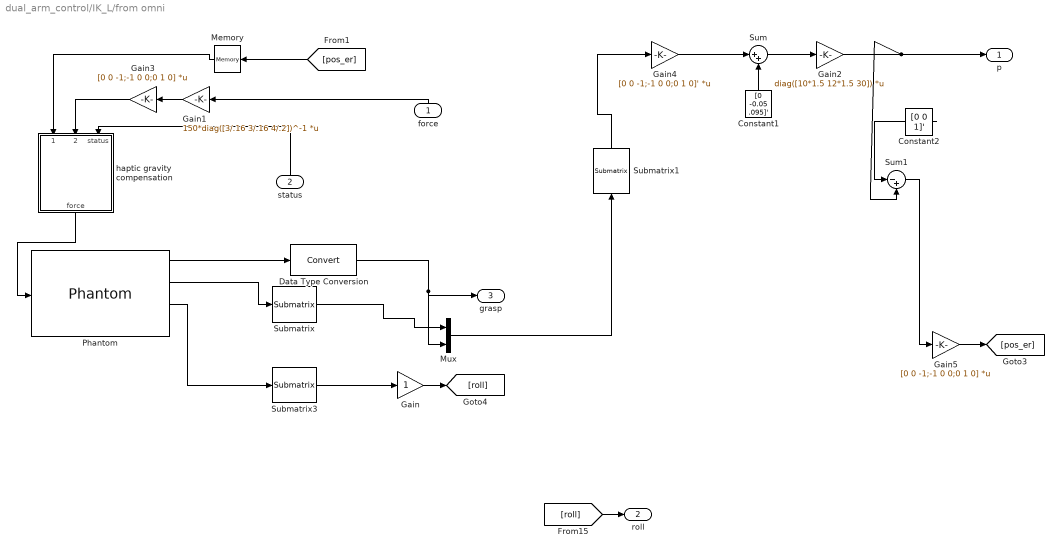
== system dual_arm_control/IK_L/from omni ==
  force : Inport
  status : Inport  Port=2
  Constant1 : Constant  Value=[0 -0.05 .095]'
  Constant2 : Constant  Value=[0 0 1]'
  Data Type Conversion : DataTypeConversion
  Gain : Gain
  Gain1 : Gain  Gain=150*diag([3/.16 3/.16 4/.2])^-1  Multiplication=Matrix(K*u)
  Gain2 : Gain  Gain=diag([10*1.5 12*1.5 30])  Multiplication=Matrix(K*u)
  Gain3 : Gain  Gain=[0 0 -1;-1 0 0;0 1 0]  Multiplication=Matrix(K*u)
  Gain4 : Gain  Gain=[0 0 -1;-1 0 0;0 1 0]'  Multiplication=Matrix(K*u)
  Gain5 : Gain  Gain=[0 0 -1;-1 0 0;0 1 0]  Multiplication=Matrix(K*u)
  Memory : Memory
  Mux : Mux  Inputs=2
  Phantom : quarc_library/Devices/Third-Party/SensAble/Phantom/Phantom  device_name=CIGITI omni  output_type=Positions and Gimbal Angles  input_type=Cartesian space  velocity_limit_option=on  velocity_limit=1200  is_7dof=off  sample_time=-1
      settings: AttributesFormatString=(%<device_name>)
  Submatrix : dspmtrx3/Submatrix  RowSpan=Range of rows  RowStartMode=First  RowStartIndex=1  RowEndMode=Index  RowEndIndex=3  ColSpan=Range of columns  ColStartMode=First  ColStartIndex=1  ColEndMode=Last  ColEndIndex=1
  Submatrix1 : dspmtrx3/Submatrix  RowSpan=Range of rows  RowStartMode=First  RowStartIndex=1  RowEndMode=Index  RowEndIndex=3  ColSpan=Range of columns  ColStartMode=First  ColStartIndex=1  ColEndMode=Last  ColEndIndex=1
  Submatrix3 : dspmtrx3/Submatrix  RowSpan=Range of rows  RowStartMode=Last  RowStartIndex=1  RowEndMode=Index  RowEndIndex=3  ColSpan=All columns  ColStartMode=First  ColStartIndex=1  ColEndMode=Last  ColEndIndex=1
  Sum : Sum  Inputs=|++
  Sum1 : Sum  Inputs=|-+
  haptic gravity compensation : Subsystem
  p : Outport
  roll : Outport  Port=2
  grasp : Outport  Port=3
  wires:
  Phantom/2 -> Submatrix/1
  Submatrix/1 -> Mux/1
  Phantom/1 -> Data Type Conversion/1
  Data Type Conversion/1 -> Mux/2, grasp/1
  Submatrix1/1 -> Gain4/1
  Constant1/1 -> Sum/2
  Sum/1 -> Gain2/1
  Gain4/1 -> Sum/1
  Mux/1 -> Submatrix1/1
  Submatrix3/1 -> Gain/1
  Phantom/3 -> Submatrix3/1
  Gain/1 -> [roll]
  Gain2/1 -> p/1, Sum1/2
  [roll] -> roll/1
  force/1 -> Gain1/1
  Memory/1 -> haptic gravity compensation/1(position)
  Gain1/1 -> Gain3/1
  Gain3/1 -> haptic gravity compensation/2(boundary force)
  [pos_er] -> Memory/1
  status/1 -> haptic gravity compensation/3(status)
  haptic gravity compensation/1(force) -> Phantom/1
  Sum1/1 -> Gain5/1
  Gain5/1 -> [pos_er]
  Constant2/1 -> Sum1/1

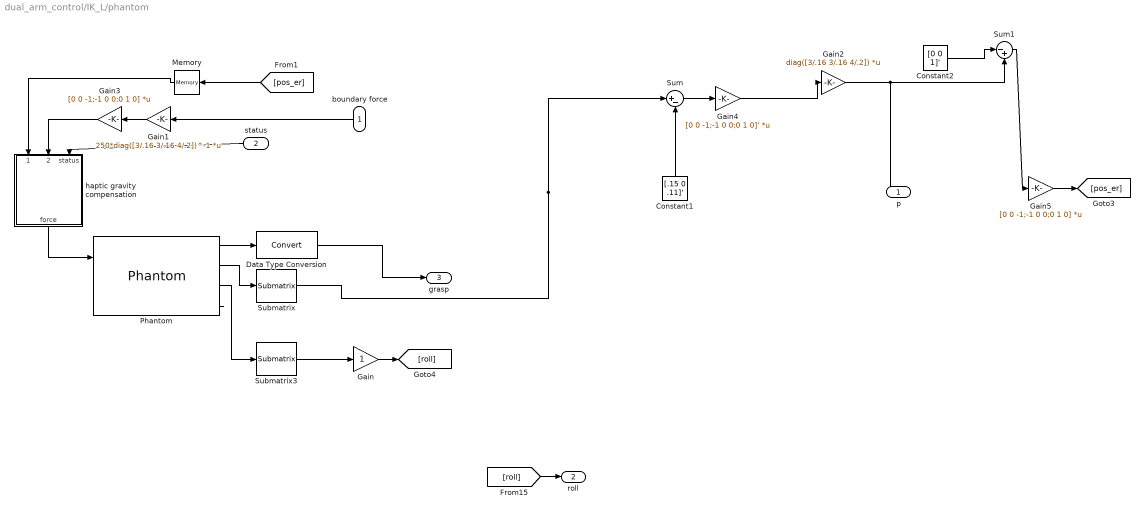
== system dual_arm_control/IK_L/phantom ==
  boundary force : Inport
  status : Inport  Port=2
  Constant1 : Constant  Value=[.15 0 .11]'
  Constant2 : Constant  Value=[0 0 1]'
  Data Type Conversion : DataTypeConversion
  Gain : Gain
  Gain1 : Gain  Gain=250*diag([3/.16 3/.16 4/.2])^-1  Multiplication=Matrix(K*u)
  Gain2 : Gain  Gain=diag([3/.16 3/.16 4/.2])  Multiplication=Matrix(K*u)
  Gain3 : Gain  Gain=[0 0 -1;-1 0 0;0 1 0]  Multiplication=Matrix(K*u)
  Gain4 : Gain  Gain=[0 0 -1;-1 0 0;0 1 0]'  Multiplication=Matrix(K*u)
  Gain5 : Gain  Gain=[0 0 -1;-1 0 0;0 1 0]  Multiplication=Matrix(K*u)
  Memory : Memory
  Phantom : quarc_library/Devices/Third-Party/SensAble/Phantom/Phantom  device_name=Default PHANToM  output_type=Positions and Gimbal Angles  input_type=Cartesian space  velocity_limit_option=on  velocity_limit=1200  is_7dof=off  sample_time=-1
      settings: AttributesFormatString=(%<device_name>)
  Submatrix : dspmtrx3/Submatrix  RowSpan=Range of rows  RowStartMode=First  RowStartIndex=1  RowEndMode=Index  RowEndIndex=3  ColSpan=Range of columns  ColStartMode=First  ColStartIndex=1  ColEndMode=Last  ColEndIndex=1
  Submatrix3 : dspmtrx3/Submatrix  RowSpan=Range of rows  RowStartMode=Last  RowStartIndex=1  RowEndMode=Index  RowEndIndex=3  ColSpan=All columns  ColStartMode=First  ColStartIndex=1  ColEndMode=Last  ColEndIndex=1
  Sum : Sum  Inputs=|+-
  Sum1 : Sum  Inputs=|-+
  haptic gravity compensation : Subsystem
  p : Outport
  roll : Outport  Port=2
  grasp : Outport  Port=3
  wires:
  Phantom/2 -> Submatrix/1
  Submatrix/1 -> Sum/1
  Phantom/1 -> Data Type Conversion/1
  Data Type Conversion/1 -> grasp/1
  Submatrix3/1 -> Gain/1
  Phantom/3 -> Submatrix3/1
  Gain/1 -> [roll]
  Gain2/1 -> p/1, Sum1/2
  Phantom/4 -> ?
  [roll] -> roll/1
  haptic gravity compensation/1(force) -> Phantom/1
  boundary force/1 -> Gain1/1
  Memory/1 -> haptic gravity compensation/1(position)
  Constant1/1 -> Sum/2
  Sum/1 -> Gain4/1
  Gain4/1 -> Gain2/1
  Gain1/1 -> Gain3/1
  Gain3/1 -> haptic gravity compensation/2(boundary force)
  [pos_er] -> Memory/1
  status/1 -> haptic gravity compensation/3(status)
  Sum1/1 -> Gain5/1
  Gain5/1 -> [pos_er]
  Constant2/1 -> Sum1/1

== system dual_arm_control/Left Arm/contoller 22 ==
  qd : Inport
  q : Inport  Port=2
  en : Inport  Port=3
  Constant : Constant  Value=15
  Constant1 : Constant  Value=1e9
  Derivative3 : Derivative
  Derivative4 : Derivative
  Derivative5 : Derivative
  Memory3 : Memory  X0="[-0.0083    0.0320    0.0169   -0.2088]'"
  slotine's adaptive : MATLAB Function  TreatAsAtomicUnit=on
  tau : Outport
  ahat : Outport  Port=2
  wires:
  Derivative4/1 -> slotine's adaptive/6(qddotdot)
  Derivative5/1 -> slotine's adaptive/8(qdot)
  Derivative3/1 -> Derivative4/1, slotine's adaptive/5(qddot)
  slotine's adaptive/2(ahat) -> Memory3/1, ahat/1
  Memory3/1 -> slotine's adaptive/9(ahat_)
  Constant/1 -> slotine's adaptive/2(lambda)
  Constant1/1 -> slotine's adaptive/3(gamma)
  qd/1 -> slotine's adaptive/4(qd), Derivative3/1
  q/1 -> slotine's adaptive/7(q), Derivative5/1
  slotine's adaptive/1(tau) -> tau/1
  en/1 -> slotine's adaptive/1(en)

== system dual_arm_control/Left Arm/controller 21 ==
  qd : Inport
  q : Inport  Port=2
  en : Inport  Port=3
  Constant : Constant  Value=100
  Constant1 : Constant  Value=1e10
  Derivative3 : Derivative
  Derivative4 : Derivative
  Derivative5 : Derivative
  Memory3 : Memory  X0="[2.4504    0.2033    0.3366    0.1727  -10.4533]'"
  slotine's adaptive : MATLAB Function  TreatAsAtomicUnit=on
  tau : Outport
  ahat : Outport  Port=2
  wires:
  Derivative4/1 -> slotine's adaptive/6(qddotdot)
  Derivative5/1 -> slotine's adaptive/8(qdot)
  Derivative3/1 -> Derivative4/1, slotine's adaptive/5(qddot)
  slotine's adaptive/2(ahat) -> Memory3/1, ahat/1
  Memory3/1 -> slotine's adaptive/9(ahat_)
  Constant/1 -> slotine's adaptive/2(lambda)
  Constant1/1 -> slotine's adaptive/3(gamma)
  qd/1 -> slotine's adaptive/4(qd), Derivative3/1
  q/1 -> slotine's adaptive/7(q), Derivative5/1
  slotine's adaptive/1(tau) -> tau/1
  en/1 -> slotine's adaptive/1(en)

== system dual_arm_control/Left Arm/controller 23 ==
  qd : Inport
  q : Inport  Port=2
  en : Inport  Port=3
  Constant : Constant  Value=90
  Constant1 : Constant  Value=1e6
  Derivative3 : Derivative
  Derivative4 : Derivative
  Derivative5 : Derivative
  Memory3 : Memory  X0="[ 2.4073    0.0972    0.0790   -5.3481]'"
  slotine's adaptive : MATLAB Function  TreatAsAtomicUnit=on
  tau : Outport
  ahat : Outport  Port=2
  wires:
  Derivative4/1 -> slotine's adaptive/6(qddotdot)
  Derivative5/1 -> slotine's adaptive/8(qdot)
  Derivative3/1 -> Derivative4/1, slotine's adaptive/5(qddot)
  slotine's adaptive/2(ahat) -> Memory3/1, ahat/1
  Memory3/1 -> slotine's adaptive/9(ahat_)
  Constant/1 -> slotine's adaptive/2(lambda)
  Constant1/1 -> slotine's adaptive/3(gamma)
  qd/1 -> slotine's adaptive/4(qd), Derivative3/1
  q/1 -> slotine's adaptive/7(q), Derivative5/1
  slotine's adaptive/1(tau) -> tau/1
  en/1 -> slotine's adaptive/1(en)

== system dual_arm_control/Left Arm/controller 24 ==
  qd : Inport
  q : Inport  Port=2
  en : Inport  Port=3
  Constant : Constant  Value=50
  Constant1 : Constant  Value=1e6
  Derivative3 : Derivative
  Derivative4 : Derivative
  Derivative5 : Derivative
  Memory3 : Memory  X0="[0.0008    0.0273    0.0390   -0.0832]'"
  slotine's adaptive : MATLAB Function  TreatAsAtomicUnit=on
  tau : Outport
  ahat : Outport  Port=2
  wires:
  Derivative4/1 -> slotine's adaptive/6(qddotdot)
  Derivative5/1 -> slotine's adaptive/8(qdot)
  Derivative3/1 -> Derivative4/1, slotine's adaptive/5(qddot)
  slotine's adaptive/2(ahat) -> Memory3/1, ahat/1
  Memory3/1 -> slotine's adaptive/9(ahat_)
  Constant/1 -> slotine's adaptive/2(lambda)
  Constant1/1 -> slotine's adaptive/3(gamma)
  qd/1 -> slotine's adaptive/4(qd), Derivative3/1
  q/1 -> slotine's adaptive/7(q), Derivative5/1
  slotine's adaptive/1(tau) -> tau/1
  en/1 -> slotine's adaptive/1(en)

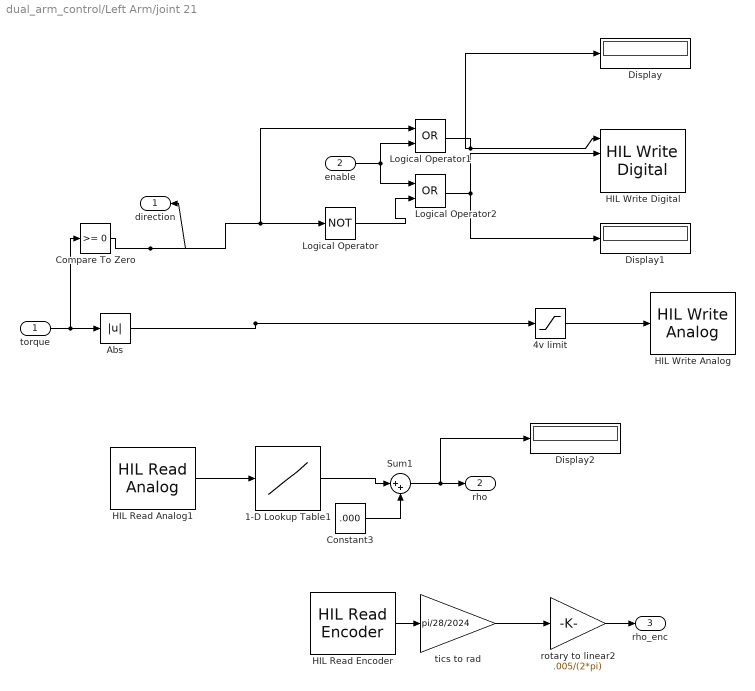
== system dual_arm_control/Left Arm/joint 21 ==
  torque : Inport
  enable : Inport  Port=2
  1-D Lookup Table1 : Lookup_n-D  NumberOfTableDimensions=1  BreakpointsForDimension1=[.14 .26 .4 .66 .92 1.21 1.59 2.49 3.63]  Table=[0.0:.005:.04]  RndMeth=Simplest  InputSameDT=on
  4v limit : Saturate  UpperLimit=4  LowerLimit=0
  Abs : Abs
  Compare To Zero : simulink/Logic and Bit Operations/Compare To Zero  relop=>=  OutDataTypeStr=boolean
  Constant3 : Constant  Value=.000
  Display : Display
  Display1 : Display
  Display2 : Display
  HIL Read Analog1 : quarc_library/Data Acquisition/Generic/Immediate I//O/HIL Read Analog  object_name=HIL-2  channels=[7]  sample_time=qc_get_step_size  active=on  vector_output=off
  HIL Read Encoder : quarc_library/Data Acquisition/Generic/Immediate I//O/HIL Read Encoder  object_name=HIL-2  channels=[4]  sample_time=qc_get_step_size  active=on  vector_output=off  data_type_mode=Inherit via back propagation  data_type=double
  HIL Write Analog : quarc_library/Data Acquisition/Generic/Immediate I//O/HIL Write Analog  object_name=HIL-1  channels=[4]  sample_time=-1  active=off  vector_input=off
  HIL Write Digital : quarc_library/Data Acquisition/Generic/Immediate I//O/HIL Write Digital  object_name=HIL-1  channels=[16:19]  sample_time=-1  active=off  vector_input=off
  Logical Operator : Logic  Operator=NOT  AllPortsSameDT=off  OutDataTypeStr=boolean
  Logical Operator1 : Logic  Operator=OR  AllPortsSameDT=off  OutDataTypeStr=boolean
  Logical Operator2 : Logic  Operator=OR  AllPortsSameDT=off  OutDataTypeStr=boolean
  Sum1 : Sum  Inputs=|++
  rotary to linear2 : Gain  Gain=.005/(2*pi)
  tics to rad : Gain  Gain=pi/28/2024
  direction : Outport
  rho : Outport  Port=2
  rho_enc : Outport  Port=3
  wires:
  4v limit/1 -> HIL Write Analog/1
  Compare To Zero/1 -> direction/1, Logical Operator/1, Logical Operator1/1
  Abs/1 -> 4v limit/1
  torque/1 -> Abs/1, Compare To Zero/1
  HIL Read Analog1/1 -> 1-D Lookup Table1/1
  Logical Operator/1 -> Logical Operator2/2
  enable/1 -> Logical Operator1/2, Logical Operator2/1
  Logical Operator1/1 -> Display/1, HIL Write Digital/1
  Logical Operator2/1 -> Display1/1, HIL Write Digital/2
  tics to rad/1 -> rotary to linear2/1
  rotary to linear2/1 -> rho_enc/1
  HIL Read Encoder/1 -> tics to rad/1
  1-D Lookup Table1/1 -> Sum1/1
  Constant3/1 -> Sum1/2
  Sum1/1 -> rho/1, Display2/1

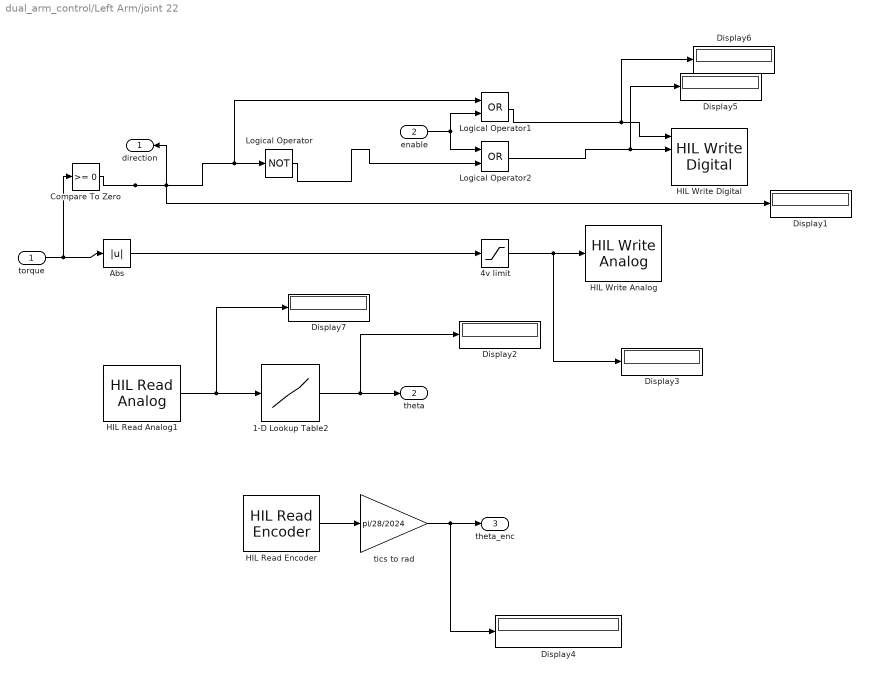
== system dual_arm_control/Left Arm/joint 22 ==
  torque : Inport
  enable : Inport  Port=2
  1-D Lookup Table2 : Lookup_n-D  NumberOfTableDimensions=1  BreakpointsForDimension1=[.06 .81 1.15 1.71 2.07 2.55 3 3.38 3.92 4.27]  Table=[2.79 2 1.58 1 .5 0 -.52 -1 -1.58 -2]  RndMeth=Simplest  InputSameDT=on
  4v limit : Saturate  UpperLimit=4  LowerLimit=0
  Abs : Abs
  Compare To Zero : simulink/Logic and Bit Operations/Compare To Zero  relop=>=  OutDataTypeStr=boolean
  Display{1..7} (7 alike) : Display
  HIL Read Analog1 : quarc_library/Data Acquisition/Generic/Immediate I//O/HIL Read Analog  object_name=HIL-1  channels=[5]  sample_time=qc_get_step_size  active=on  vector_output=off
  HIL Read Encoder : quarc_library/Data Acquisition/Generic/Immediate I//O/HIL Read Encoder  object_name=HIL-2  channels=[5]  sample_time=qc_get_step_size  active=on  vector_output=off  data_type_mode=Inherit via back propagation  data_type=double
  HIL Write Analog : quarc_library/Data Acquisition/Generic/Immediate I//O/HIL Write Analog  object_name=HIL-1  channels=[5]  sample_time=-1  active=off  vector_input=off
  HIL Write Digital : quarc_library/Data Acquisition/Generic/Immediate I//O/HIL Write Digital  object_name=HIL-1  channels=[20:23]  sample_time=-1  active=off  vector_input=off
  Logical Operator : Logic  Operator=NOT  AllPortsSameDT=off  OutDataTypeStr=boolean
  Logical Operator1 : Logic  Operator=OR  AllPortsSameDT=off  OutDataTypeStr=boolean
  Logical Operator2 : Logic  Operator=OR  AllPortsSameDT=off  OutDataTypeStr=boolean
  tics to rad : Gain  Gain=pi/28/2024
  direction : Outport
  theta : Outport  Port=2
  theta_enc : Outport  Port=3
  wires:
  4v limit/1 -> HIL Write Analog/1, Display3/1
  Compare To Zero/1 -> Logical Operator/1, Logical Operator1/1, direction/1, Display1/1
  Abs/1 -> 4v limit/1
  torque/1 -> Abs/1, Compare To Zero/1
  HIL Read Analog1/1 -> 1-D Lookup Table2/1, Display7/1
  HIL Read Encoder/1 -> tics to rad/1
  Logical Operator/1 -> Logical Operator2/2
  Logical Operator1/1 -> HIL Write Digital/1, Display6/1
  Logical Operator2/1 -> HIL Write Digital/2, Display5/1
  enable/1 -> Logical Operator1/2, Logical Operator2/1
  tics to rad/1 -> theta_enc/1, Display4/1
  1-D Lookup Table2/1 -> Display2/1, theta/1

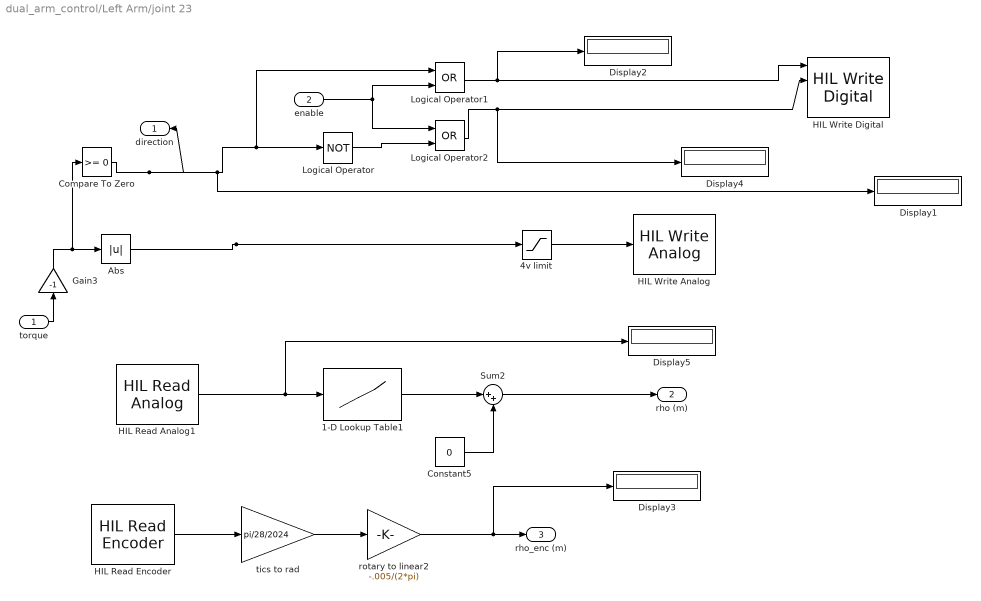
== system dual_arm_control/Left Arm/joint 23 ==
  torque : Inport
  enable : Inport  Port=2
  1-D Lookup Table1 : Lookup_n-D  NumberOfTableDimensions=1  BreakpointsForDimension1=[.11 .2 .36 .63 .88 1.15 1.52 2.26 3.43]  Table=[.04 .035 .03 .025 .02 .015 .01 .005 0]  RndMeth=Simplest  InputSameDT=on
  4v limit : Saturate  UpperLimit=4  LowerLimit=0
  Abs : Abs
  Compare To Zero : simulink/Logic and Bit Operations/Compare To Zero  relop=>=  OutDataTypeStr=boolean
  Constant5 : Constant  Value=0
  Display{1..5} (5 alike) : Display
  Gain3 : Gain  Gain=-1
  HIL Read Analog1 : quarc_library/Data Acquisition/Generic/Immediate I//O/HIL Read Analog  object_name=HIL-2  channels=[6]  sample_time=qc_get_step_size  active=on  vector_output=off
  HIL Read Encoder : quarc_library/Data Acquisition/Generic/Immediate I//O/HIL Read Encoder  object_name=HIL-2  channels=[6]  sample_time=qc_get_step_size  active=on  vector_output=off  data_type_mode=Inherit via back propagation  data_type=double
  HIL Write Analog : quarc_library/Data Acquisition/Generic/Immediate I//O/HIL Write Analog  object_name=HIL-1  channels=[6]  sample_time=-1  active=off  vector_input=off
  HIL Write Digital : quarc_library/Data Acquisition/Generic/Immediate I//O/HIL Write Digital  object_name=HIL-1  channels=[24:27]  sample_time=-1  active=off  vector_input=off
  Logical Operator : Logic  Operator=NOT  AllPortsSameDT=off  OutDataTypeStr=boolean
  Logical Operator1 : Logic  Operator=OR  AllPortsSameDT=off  OutDataTypeStr=boolean
  Logical Operator2 : Logic  Operator=OR  AllPortsSameDT=off  OutDataTypeStr=boolean
  Sum2 : Sum  Inputs=|++
  rotary to linear2 : Gain  Gain=-.005/(2*pi)
  tics to rad : Gain  Gain=pi/28/2024
  direction : Outport
  rho (m) : Outport  Port=2
  rho_enc (m) : Outport  Port=3
  wires:
  4v limit/1 -> HIL Write Analog/1
  Compare To Zero/1 -> direction/1, Logical Operator1/1, Logical Operator/1, Display1/1
  Abs/1 -> 4v limit/1
  torque/1 -> Gain3/1
  HIL Read Encoder/1 -> tics to rad/1
  ? -> ?
  Logical Operator1/1 -> Display2/1, HIL Write Digital/1
  Logical Operator2/1 -> Display4/1, HIL Write Digital/2
  enable/1 -> Logical Operator1/2, Logical Operator2/1
  tics to rad/1 -> rotary to linear2/1
  rotary to linear2/1 -> rho_enc (m)/1, Display3/1
  HIL Read Analog1/1 -> 1-D Lookup Table1/1, Display5/1
  1-D Lookup Table1/1 -> Sum2/1
  Constant5/1 -> Sum2/2
  Sum2/1 -> rho (m)/1
  Logical Operator/1 -> Logical Operator2/2
  Gain3/1 -> Abs/1, Compare To Zero/1

== system dual_arm_control/Left Arm/joint 24 ==
  torque : Inport
  enable : Inport  Port=2
  1-D Lookup Table3 : Lookup_n-D  NumberOfTableDimensions=1  BreakpointsForDimension1=[.94 1.45 2.23 3.02 3.52]  Table=[pi/2 1 0 -1 -pi/2]  RndMeth=Simplest  InputSameDT=on
  4v limit : Saturate  UpperLimit=4  LowerLimit=0
  Abs : Abs
  Compare To Zero : simulink/Logic and Bit Operations/Compare To Zero  relop=>=  OutDataTypeStr=boolean
  Display2 : Display
  Display6 : Display
  HIL Read Analog1 : quarc_library/Data Acquisition/Generic/Immediate I//O/HIL Read Analog  object_name=HIL-1  channels=[7]  sample_time=qc_get_step_size  active=on  vector_output=off
  HIL Read Encoder : quarc_library/Data Acquisition/Generic/Immediate I//O/HIL Read Encoder  object_name=HIL-2  channels=[7]  sample_time=qc_get_step_size  active=on  vector_output=off  data_type_mode=Inherit via back propagation  data_type=double
  HIL Write Analog : quarc_library/Data Acquisition/Generic/Immediate I//O/HIL Write Analog  object_name=HIL-1  channels=[7]  sample_time=-1  active=off  vector_input=off
  HIL Write Digital : quarc_library/Data Acquisition/Generic/Immediate I//O/HIL Write Digital  object_name=HIL-1  channels=[28:31]  sample_time=-1  active=off  vector_input=off
  Logical Operator : Logic  Operator=NOT  AllPortsSameDT=off  OutDataTypeStr=boolean
  Logical Operator1 : Logic  Operator=OR  AllPortsSameDT=off  OutDataTypeStr=boolean
  Logical Operator2 : Logic  Operator=OR  AllPortsSameDT=off  OutDataTypeStr=boolean
  tics to rad : Gain  Gain=pi/28/2024
  theta_enc : Outport
  theta : Outport  Port=2
  wires:
  4v limit/1 -> HIL Write Analog/1, Display2/1
  Compare To Zero/1 -> Logical Operator/1, Logical Operator1/1
  Abs/1 -> 4v limit/1
  torque/1 -> Compare To Zero/1, Abs/1
  Logical Operator1/1 -> HIL Write Digital/1
  Logical Operator2/1 -> HIL Write Digital/2
  HIL Read Encoder/1 -> tics to rad/1
  HIL Read Analog1/1 -> Display6/1, 1-D Lookup Table3/1
  tics to rad/1 -> theta_enc/1
  enable/1 -> Logical Operator1/2, Logical Operator2/1
  Logical Operator/1 -> Logical Operator2/2
  1-D Lookup Table3/1 -> theta/1

== system dual_arm_control/Right Arm/M14 ==
  torque : Inport
  enable : Inport  Port=2
  1-D Lookup Table3 : Lookup_n-D  NumberOfTableDimensions=1  BreakpointsForDimension1=[1.83 2.47 3.11 3.43 4.14 ]  Table=[-pi/2 -pi/4 0 pi/4 pi/2]  RndMeth=Simplest  InputSameDT=on
  4v limit : Saturate  UpperLimit=4  LowerLimit=0
  Abs : Abs
  Compare To Zero : simulink/Logic and Bit Operations/Compare To Zero  relop=>=  OutDataTypeStr=boolean
  Display : Display
  HIL Read Analog1 : quarc_library/Data Acquisition/Generic/Immediate I//O/HIL Read Analog  object_name=HIL-1  channels=[3]  sample_time=qc_get_step_size  active=on  vector_output=off
  HIL Read Encoder : quarc_library/Data Acquisition/Generic/Immediate I//O/HIL Read Encoder  object_name=HIL-2  channels=[3]  sample_time=qc_get_step_size  active=on  vector_output=off  data_type_mode=Inherit via back propagation  data_type=double
  HIL Write Analog : quarc_library/Data Acquisition/Generic/Immediate I//O/HIL Write Analog  object_name=HIL-1  channels=[3]  sample_time=-1  active=off  vector_input=off
  HIL Write Digital : quarc_library/Data Acquisition/Generic/Immediate I//O/HIL Write Digital  object_name=HIL-1  channels=[12:15]  sample_time=-1  active=off  vector_input=off
  Logical Operator : Logic  Operator=NOT  AllPortsSameDT=off  OutDataTypeStr=boolean
  Logical Operator1 : Logic  Operator=OR  AllPortsSameDT=off  OutDataTypeStr=boolean
  Logical Operator2 : Logic  Operator=OR  AllPortsSameDT=off  OutDataTypeStr=boolean
  tics to rad : Gain  Gain=pi/28/2024
  direction : Outport
  theta : Outport  Port=2
  theta_enc : Outport  Port=3
  wires:
  4v limit/1 -> HIL Write Analog/1
  Compare To Zero/1 -> direction/1, Logical Operator/1, Logical Operator1/1
  Abs/1 -> 4v limit/1
  torque/1 -> Abs/1, Compare To Zero/1
  HIL Read Analog1/1 -> 1-D Lookup Table3/1
  HIL Read Encoder/1 -> tics to rad/1
  Logical Operator/1 -> Logical Operator2/2
  Logical Operator1/1 -> HIL Write Digital/1
  enable/1 -> Logical Operator1/2, Logical Operator2/1
  Logical Operator2/1 -> HIL Write Digital/2
  tics to rad/1 -> theta_enc/1
  1-D Lookup Table3/1 -> theta/1, Display/1
